simulink model "ProbOne"  (R2020b)
settings: Solver=VariableStepAuto  StartTime=0.0  StopTime=inf  RelTol=1e-3
libraries: commutil2 x1
settings Model: EnablePacing=on  Creator=vigne  LastModifiedBy='Z'ome

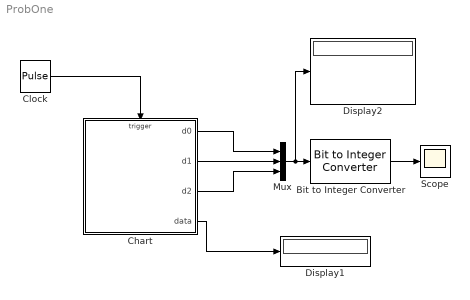
== system ProbOne ==
  Bit to Integer Converter : commutil2/Bit to Integer Converter  nbits=3  bitOrder=LSB first  signedOutputValues=Unsigned  outDtype=Inherit via internal rule  outDtypeSigned=Inherit via internal rule
  Chart : Stateflow chart  TreatAsAtomicUnit=on
  Clock : DiscretePulseGenerator  PulseType=Time based  Period=0.5  PulseWidth=5
  Display1 : Display
  Display2 : Display
  Mux : Mux  Inputs=3
  Scope : Scope
  wires:
  Mux/1 -> Display2/1, Bit to Integer Converter/1
  Chart/1(d0) -> Mux/1
  Chart/2(d1) -> Mux/2
  Chart/3(d2) -> Mux/3
  Clock/1 -> Chart/Trigger
  Chart/4(data) -> Display1/1
  Bit to Integer Converter/1 -> Scope/1

== stateflow chart ProbOne/Chart ==
  state ConversionState [parallel]
    during:
    data2=d2;
    data1=d1;
    data0=d0;
    r=0;
    check(data2,data1,data0);
    settings: executionOrder=4
  state digit0 [parallel]
    settings: executionOrder=1
    state zero
      en:
      d0=0;
    state one
      en:
      d0=1
    digit0.zero -> digit0.zero [order 2] : [pulse && reset]
    digit0.one -> digit0.zero [order 2] : reset
    (default) -> digit0.zero
    digit0.one -> digit0.zero [order 1] : pulse{send(inc1);}
    digit0.zero -> digit0.one [order 1] : pulse
  note: 000-0
      | 001-1
      | 010-2
      | 011-3
      | 100-4
      | 101-5
      | 110-6
      | 111-7
  state check(d02,d01,d00) [function]
    (default) -> (junction 123) : % Conversion to Decimal
    (junction 123) -> (junction 128) [order 1] : [d02==0 && d01==0 && d00==0]
    (junction 123) -> (junction 124) [order 2]
    (junction 128) -> (junction 150) : {data=0;
        | r=0;}
    (junction 124) -> (junction 126) [order 1] : [d02==0 && d01==0 && d00==1]
    (junction 124) -> (junction 127) [order 2]
    (junction 126) -> (junction 137) : {data=1;
        | r=0;}
    (junction 127) -> (junction 125) [order 1] : [d02==0 && d01==1 && d00==0]
    (junction 127) -> (junction 129) [order 2]
    (junction 125) -> (junction 131) : {data=2;
        | r=0;}
    (junction 129) -> (junction 134) [order 1] : [d02==0 && d01==1 && d00==1]
    (junction 129) -> (junction 187) [order 2]
    (junction 134) -> (junction 133) : {data=3;
        | r=0;}
    (junction 187) -> (junction 132) [order 1] : [d02==1 && d01==0 && d00==0]
    (junction 187) -> (junction 193) [order 2]
    (junction 132) -> (junction 136) : {data=4;
        | r=0;}
    (junction 193) -> (junction 195) [order 1] : [d02==1 && d01==0 && d00==1 && pulse]
    (junction 193) -> (junction 130) [order 2]
    (junction 195) -> (junction 196) : {send(reset)}
    (junction 196) -> (junction 130)
    (junction 136) -> (junction 196)
    (junction 133) -> (junction 136)
    (junction 131) -> (junction 133)
    (junction 137) -> (junction 131)
    (junction 150) -> (junction 137)
    (junction 130) -> (junction 143)
  state digit1 [parallel]
    settings: executionOrder=2
    state zero
      en:
      d1=0;
    state one
      en:
      d1=1;
    digit1.one -> digit1.zero [order 2] : reset
    (default) -> digit1.zero
    digit1.one -> digit1.zero [order 1] : inc1{send(inc2);}
    digit1.zero -> digit1.one : inc1
  state digit2 [parallel]
    settings: executionOrder=3
    state zero
      en:
      d2=0;
    state one
      en:
      d2=1;
    digit2.one -> digit2.zero [order 2] : reset
    (default) -> digit2.zero
    digit2.one -> digit2.zero [order 1] : inc2
    digit2.zero -> digit2.one : inc2
  (default) -> digit0
  data: d02 function_input; d01 function_input; d00 function_input; d0 output; d1 output; d2 output; data output; data0 local; data1 local; data2 local; r local
  events: pulse input RISING_EDGE_EVENT; inc1 local FUNCTION_CALL_EVENT; inc2 local FUNCTION_CALL_EVENT; reset local EITHER_EDGE_EVENT
